simulink model "ball_simulation"  (Simulink 6.3)
settings: Solver=ode45  StartTime=0.0  StopTime=20.0  RelTol=1e-3
settings Model: LastModifiedBy=Ms1

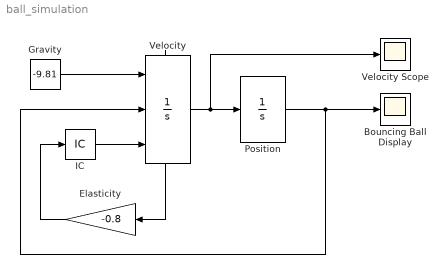
== system ball_simulation ==
  Bouncing Ball Display : Scope
  Elasticity : Gain  Orientation=left  Gain=-0.8  SaturateOnIntegerOverflow=on
  Gravity : Constant  Value=-9.81
  IC : InitialCondition  Value=15
  Position : Integrator  InitialCondition=10  LimitOutput=on  LowerSaturationLimit=0
  Velocity : Integrator  ExternalReset=falling  InitialConditionSource=external  ShowStatePort=on
  Velocity Scope : Scope
  wires:
  Gravity/1 -> Velocity/1
  IC/1 -> Velocity/3
  Velocity/1 -> Position/1, Velocity Scope/1
  Position/1 -> Bouncing Ball Display/1, Velocity/2
  Velocity/State -> Elasticity/1
  Elasticity/1 -> IC/1
